simulink model "mux4_1_model"  (R2023b)
settings: Solver=VariableStepAuto  StartTime=0.0  StopTime=10.0  RelTol=1e-3
libraries: neural x204
(part 4 of 4)

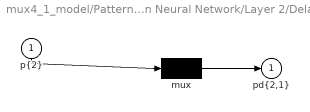
== system mux4_1_model/Pattern Recognition Neural Network/Layer 2/Delays 1 ==
  "p{2}" : Inport  PortDimensions=200
      mask Display: e = 0.06;c1 = [120 230 180]/255;c2 = ([120 230 180]+0)/(256+128);c3 = ([120 230 180]+128)/(256+128);patch([0 1 1 0],[0 0 1 1],c1);patch([0 1 1 1-e 1-e 0+e],[0 0 1 1-e 0+e 0+e],c2);patch([0 0 1 1-e 0+e 0+e],[0 1 1 1-e 1-e 0+e],c3);plot([0 1 1 0 0],[0 0 1 1 0]);
  mux : Mux  Inputs=1
      mask Display: e = 0.06;c1 = [120 150 230]/255;c2 = ([120 150 230]+0)/383;c3 = ([120 150 230]+128)/383;patch([0 1 1 0],[0 0 1 1],c1);patch([0 1 1 1-e 1-e 0+e],[0 0 1 1-e 0+e 0+e],c2);patch([0 0 1 1-e 0+e 0+e],[0 1 1 1-e 1-e 0+e],c3);plot([0 1 1 0 0],[0 0 1 1 0]);disp('Mux')
  "pd{2,1}" : Outport
      mask Display: e = 0.06;c1 = [120 230 180]/255;c2 = ([120 230 180]+0)/(256+128);c3 = ([120 230 180]+128)/(256+128);patch([0 1 1 0],[0 0 1 1],c1);patch([0 1 1 1-e 1-e 0+e],[0 0 1 1-e 0+e 0+e],c2);patch([0 0 1 1-e 0+e 0+e],[0 1 1 1-e 1-e 0+e],c3);plot([0 1 1 0 0],[0 0 1 1 0]);
  wires:
  "p{2}"/1 -> mux/1
  mux/1 -> "pd{2,1}"/1

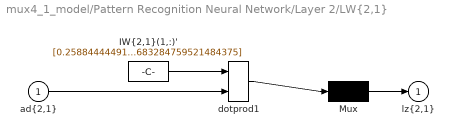
== system mux4_1_model/Pattern Recognition Neural Network/Layer 2/LW{2,1} ==
  "ad{2,1}" : Inport  PortDimensions=200
      mask Display: e = 0.06;c1 = [120 230 180]/255;c2 = ([120 230 180]+0)/(256+128);c3 = ([120 230 180]+128)/(256+128);patch([0 1 1 0],[0 0 1 1],c1);patch([0 1 1 1-e 1-e 0+e],[0 0 1 1-e 0+e 0+e],c2);patch([0 0 1 1-e 0+e 0+e],[0 1 1 1-e 1-e 0+e],c3);plot([0 1 1 0 0],[0 0 1 1 0]);
  "IW{2,1}(1,:)'" : Constant  Value=[0.2588444449145708148307676310651004314422607421875;-0.2020408538202399240102380417738459073007106781005859375;0.69703092863651361366095215998939238488674163818359375;0.902719171018663502081835758872330188751220703125;-0.163315265726805047830083594817551784217357635498046875;-1.17921062502983886588481254875659942626953125;1.2456176142150621188875447842292487621307373046875;0.11879546885841228698321714318808517418801784515380859375;0.42584328992150910497826998835080303251743316650390625;0.2101369043561073512993431222639628686010837554931640625;0.11353139343531902516470921682412154041230678558349609375;0.21824388534486960367075880640186369419097900390625;-0.45068247288516805060254455383983440697193145751953125;-0.54083501272788059299756469044950790703296661376953125;-0.001153167074947003545304369254154153168201446533203125;-0.75525023019355985720579838016419671475887298583984375;-1.0275246086257203703695495278225280344486236572265625;-0.269384708862355548575351349427364766597747802734375;0.405034519581895124940018604320357553660869598388671875;-0.5720229924991644399057122427620925009250640869140625;0.9973278293338989630711921563488431274890899658203125;0.417314873487164728071974195700022391974925994873046875;1.576521222148838052845576385152526199817657470703125;-0.46597963806427766808582191515597514808177947998046875;0.63950649132625991821754496413632296025753021240234375;-0.67441199154104281010546628749580122530460357666015625;0.292892769719726053789798925208742730319499969482421875;-0.6517062428543425323113069680402986705303192138671875;-0.70345912366845697594186503920354880392551422119140625;0.1759063278865482249369023293184000067412853240966796875;-0.433383323542506193604140207753516733646392822265625;0.400558637992469768196457380327046848833560943603515625;-0.3386866623913273866008921686443500220775604248046875;0.783742786920948564244326917105354368686676025390625;-0.57020018887959411646448870669701136648654937744140625;-0.263780252642639378990452314610593020915985107421875;-0.5472511747182500219111034311936236917972564697265625;-0.2031447167167391987252500484828487969934940338134765625;-0.2099527251224580781663320294683217070996761322021484375;-1.093097862741867487557101412676274776458740234375;-0.2975620089595789607983533642254769802093505859375;0.39215628123235812818592194162192754447460174560546875;-0.6134513735238027454244047476095147430896759033203125;0.62087600334916592803580215331749059259891510009765625;-0.5295716934902812145224970663548447191715240478515625;0.878727756416046279497322757379151880741119384765625;0.3937392151062883982604034827090799808502197265625;1.288372800530481754321954213082790374755859375;-0.8326995178771394723327148312819190323352813720703125;-0.00458911251034709033458369731306447647511959075927734375;0.427519301957803465885632476783939637243747711181640625;0.1877314183271258929419644800873356871306896209716796875;0.04717124806679862114577872489462606608867645263671875;-0.01459935699232954055271083149136757128871977329254150390625;0.392225204852593545279404452230664901435375213623046875;-0.378854842962597249123035680895554833114147186279296875;-0.258649150013272877135506178092327900230884552001953125;0.3544323983183754744885618492844514548778533935546875;-0.2016897037544781168261209813863388262689113616943359375;-0.3184780136587022081329223510692827403545379638671875;0.157750324667830454927752725780010223388671875;-0.6280616312679330182078274447121657431125640869140625;0.64236651182768789158927802418475039303302764892578125;0.356585733512457425664621268879272975027561187744140625;0.932469374079399671018109074793756008148193359375;-1.1129358466845713504511650171480141580104827880859375;-0.399488694002560651430400184835889376699924468994140625;-0.35784102170635068151938185110338963568210601806640625;-0.11071498507486686457834679231382324360311031341552734375;0.366553923894113342640821429085917770862579345703125;1.1406367302462478985347615889622829854488372802734375 ...(+7246 chars)]
      mask Display: e = 0.06;c1 = [120 150 230]/255;c2 = ([120 150 230]+0)/383;c3 = ([120 150 230]+128)/383;patch([0 1 1 0],[0 0 1 1],c1);patch([0 1 1 1-e 1-e 0+e],[0 0 1 1-e 0+e 0+e],c2);patch([0 0 1 1-e 0+e 0+e],[0 1 1 1-e 1-e 0+e],c3);plot([0 1 1 0 0],[0 0 1 1 0]);disp('weights');
  Mux : Mux  Inputs=1
      mask Display: e = 0.06;c1 = [120 150 230]/255;c2 = ([120 150 230]+0)/383;c3 = ([120 150 230]+128)/383;patch([0 1 1 0],[0 0 1 1],c1);patch([0 1 1 1-e 1-e 0+e],[0 0 1 1-e 0+e 0+e],c2);patch([0 0 1 1-e 0+e 0+e],[0 1 1 1-e 1-e 0+e],c3);plot([0 1 1 0 0],[0 0 1 1 0]);disp('Mux');
  dotprod1 : neural/Weight Functions/dotprod
  "lz{2,1}" : Outport
      mask Display: e = 0.06;c1 = [120 230 180]/255;c2 = ([120 230 180]+0)/(256+128);c3 = ([120 230 180]+128)/(256+128);patch([0 1 1 0],[0 0 1 1],c1);patch([0 1 1 1-e 1-e 0+e],[0 0 1 1-e 0+e 0+e],c2);patch([0 0 1 1-e 0+e 0+e],[0 1 1 1-e 1-e 0+e],c3);plot([0 1 1 0 0],[0 0 1 1 0]);
  wires:
  "IW{2,1}(1,:)'"/1 -> dotprod1/1
  "ad{2,1}"/1 -> dotprod1/2
  dotprod1/1 -> Mux/1
  Mux/1 -> "lz{2,1}"/1
